simulink model "LONG_accn"  (R2015a)
settings: Solver=ode45  StartTime=0.0  StopTime=10.0  RelTol=1e-3
undefined symbols (not defined in the file): m
settings Model: Creator=BML  LastModifiedBy=BML

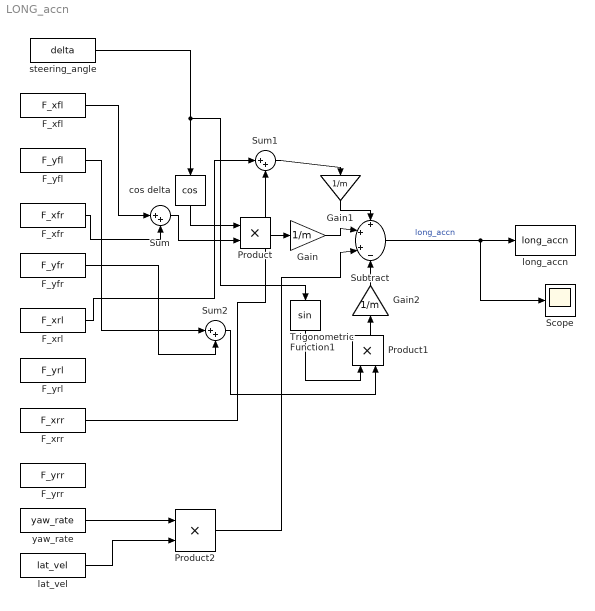
== system LONG_accn ==
  F_xfl : FromWorkspace  VariableName=F_xfl  SampleTime=0
  F_xfr : FromWorkspace  VariableName=F_xfr  SampleTime=0
  F_xrl : FromWorkspace  VariableName=F_xrl  SampleTime=0
  F_xrr : FromWorkspace  VariableName=F_xrr  SampleTime=0
  F_yfl : FromWorkspace  VariableName=F_yfl  SampleTime=0
  F_yfr : FromWorkspace  VariableName=F_yfr  SampleTime=0
  F_yrl : FromWorkspace  VariableName=F_yrl  SampleTime=0
  F_yrr : FromWorkspace  VariableName=F_yrr  SampleTime=0
  Gain : Gain  Gain=1/m
  Gain1 : Gain  Gain=1/m
  Gain2 : Gain  Gain=1/m
  Product : Product
  Product1 : Product
  Product2 : Product
  Scope : Scope
  Subtract : Sum  Inputs=+++-
  Sum : Sum  Inputs=|++
  Sum1 : Sum  Inputs=|++
  Sum2 : Sum  Inputs=|++
  Trigonometric Function1 : Trigonometry
  cos delta : Trigonometry  Operator=cos
  lat_vel : FromWorkspace  VariableName=lat_vel  SampleTime=0
  long_accn : ToWorkspace  VariableName=long_accn  SaveFormat=Timeseries  SampleTime=-1
  steering_angle : FromWorkspace  VariableName=delta  SampleTime=0
  yaw_rate : FromWorkspace  VariableName=yaw_rate  SampleTime=0
  wires:
  Product2/1 -> Subtract/3
  Gain/1 -> Subtract/2
  cos delta/1 -> Product/1
  Sum/1 -> Product/2
  Product/1 -> Gain/1
  Gain1/1 -> Subtract/1
  F_xfl/1 -> Sum/1
  F_xfr/1 -> Sum/2
  Sum1/1 -> Gain1/1
  F_xrl/1 -> Sum1/1
  F_xrr/1 -> Sum1/2
  lat_vel/1 -> Product2/2
  F_yfl/1 -> Sum2/1
  F_yfr/1 -> Sum2/2
  steering_angle/1 -> Trigonometric Function1/1, cos delta/1
  Trigonometric Function1/1 -> Product1/1
  Sum2/1 -> Product1/2
  Product1/1 -> Gain2/1
  Gain2/1 -> Subtract/4
  Subtract/1 -> Scope/1, long_accn/1  "long_accn"
  yaw_rate/1 -> Product2/1
